simulink model "untitled6"  (R2016a)
settings: Solver=VariableStepAuto  StartTime=0.0  StopTime=0.02  MaxStep=1e-6  RelTol=1e-3
libraries: powerlib x10, simulink x1
settings Model: Creator=lenovo  LastModifiedBy=lenovo

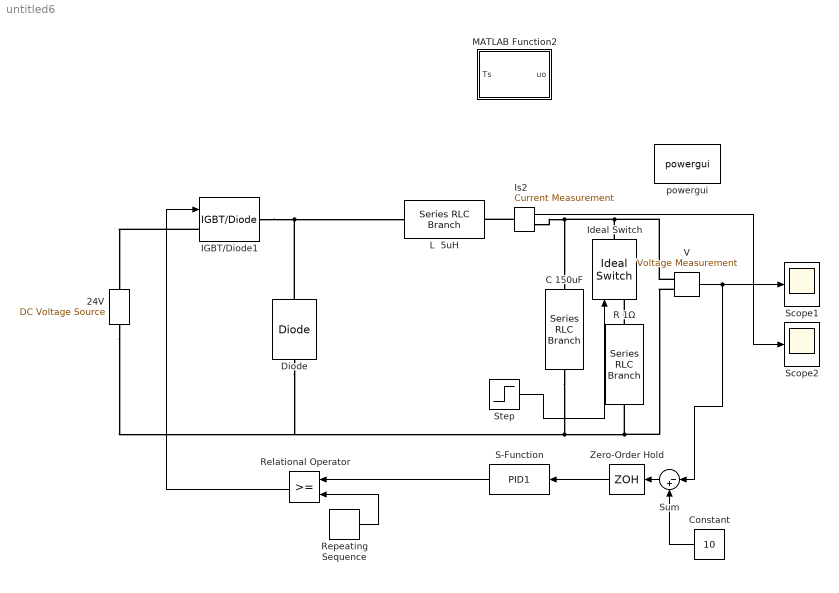
== system untitled6 ==
  24V : powerlib/Electrical Sources/DC Voltage Source  Amplitude=24  Measurements=None
  C 150uF : powerlib/Elements/Series RLC Branch  LConnTagsString=__new0  RConnTagsString=__new0  BranchType=C  Resistance=1  Inductance=1e-3  SetiL0=off  InitialCurrent=0  Capacitance=150e-6  Setx0=off  InitialVoltage=0  Measurements=None
  Constant : Constant  Value=10
  Diode : powerlib/Power Electronics/Diode  Ron=0.001  Lon=0  Vf=0.8  IC=0  UseSnubber=off  Rs=500  Cs=250e-9  Measurements=off
  IGBT/Diode1 : powerlib/Power Electronics/IGBT//Diode  Ron=1e-3  Rs=1e5  Cs=inf  Measurements=off
  Ideal Switch : powerlib/Power Electronics/Ideal Switch  Ron=0.001  Lon=0  IC=0  Rs=1  Cs=inf  Measurements=off
  Is2 : powerlib/Measurements/Current Measurement  PhasorSimulation=off  OutputType=Complex  PSBequivalent=0
  L  5uH : powerlib/Elements/Series RLC Branch  LConnTagsString=__new0  RConnTagsString=__new0  BranchType=L  Resistance=1  Inductance=5e-6  SetiL0=off  InitialCurrent=0  Capacitance=1e-6  Setx0=off  InitialVoltage=0  Measurements=None
  MATLAB Function2 : MATLAB Function  TreatAsAtomicUnit=on
  R 1Ω : powerlib/Elements/Series RLC Branch  LConnTagsString=__new0  RConnTagsString=__new0  BranchType=R  Resistance=1  Inductance=1e-3  SetiL0=off  InitialCurrent=0  Capacitance=1e-6  Setx0=off  InitialVoltage=0  Measurements=None
  Relational Operator : RelationalOperator  OutDataTypeStr=boolean
  Repeating Sequence : simulink/Sources/Repeating Sequence  rep_seq_t=[0 1e-5 2e-5]  rep_seq_y=[0.9 3.3 0.9]
  S-Function : S-Function  FunctionName=PID1  Parameters=0.0385 0.03392  SFunctionDeploymentMode=off  EnableBusSupport=off
  Scope1 : Scope
  Scope2 : Scope
  Step : Step  Time=0.01  SampleTime=0
  Sum : Sum  Inputs=|-+
  V : powerlib/Measurements/Voltage Measurement  PhasorSimulation=off  OutputType=Complex  PSBequivalent=0
  Zero-Order Hold : ZeroOrderHold  SampleTime=1e-5
  powergui : powerlib/powergui  Priority=1  SimulationMode=Continuous  SolverType=Tustin/Backward Euler (TBE)  SampleTime=1e-5  frequency=60  SPID=off  DisableSnubberDevices=off  DisableRonSwitches=off  DisableVfSwitches=off  SwTol=0  DisplayEquations=off  Interpol=off  ExternalGateDelay=off  methode=off  Ts=10  FunctionMessages=off  echomessages=off  HookPort=off  EnableUseOfTLC=off  x0status=blocks  frequencyindice=0  Pbase=100e6  ErrMax=1e-4  Iterations=50  UnitsV=kV  UnitsW=MW  buscounter=0  RestoreLinks=warning  ResistiveCurrentMeasurement=off  Frange=[0:2:500]  Ylog=off  Xlog=on  ShowGrid=off  save=off  variable=ZData  structure=0  ZoomFFT=off  StartTime=0.0  cycles=1  DisplayStyle=1  fundamental=60  FreqAxis=off  MaxFrequency=1000  frequencyindicesteady=1  RmsSteady=1  display=off
  wires:
  Repeating Sequence/1 -> Relational Operator/2
  Relational Operator/1 -> IGBT/Diode1/1
  Step/1 -> Ideal Switch/1
  Zero-Order Hold/1 -> S-Function/1
  S-Function/1 -> Relational Operator/1
  V/1 -> Sum/1, Scope1/1
  Constant/1 -> Sum/2
  Sum/1 -> Zero-Order Hold/1
  Is2/1 -> Scope2/1
  connections:
  V/LConn1 -- Ideal Switch/RConn1 -- Is2/RConn1 -- C 150uF/LConn1
  C 150uF/RConn1 -- Diode/LConn1 -- 24V/LConn1 -- V/LConn2 -- R 1Ω/RConn1
  IGBT/Diode1/RConn1 -- Diode/RConn1 -- L  5uH/LConn1
  IGBT/Diode1/LConn1 -- 24V/RConn1
  Is2/LConn1 -- L  5uH/RConn1
  R 1Ω/LConn1 -- Ideal Switch/LConn1

== matlab function untitled6/MATLAB Function2 ==
  data: uo input; Ts output
function Ts = fcn(uo)
if isempty(uo)
    uo=0;
end
persistent Uref
Uref=10;
persistent e1 e2 e3 y1 y2 y3;
if isempty(e1)
    e1=0;
end
if isempty(e2)
    e2=0;
end
if isempty(y1)
    y1=0;
end
if isempty(y2)
    y2=0;
end
e3=Uref-uo;
y3=1.285*y2-0.2847*y1+0.08191*e3-0.117*e2+0.0418*e1;
Ts=y2;
e1=e2;
e2=e3;
y1=y2;
y2=y3;
